simulink model "sf_ttable"  (R2015b)
settings: Solver=ode45  StartTime=0.0  StopTime=10  RelTol=1e-3
settings Model: Creator=amatsumo  LastModifiedBy=amatsumo
settings DataIOCC: SaveFormat=Array  SignalLoggingSaveFormat=ModelDataLogs
settings OptimizationCC: BlockReduction=off  ConditionallyExecuteInputs=off  ExpressionDepthLimit=2147483647
settings DebuggingCC: UnderspecifiedInitializationDetection=Classic  MergeDetectMultiDrivingBlocksExec=none  SolverPrmCheckMsg=warning  FcnCallInpInsideContextMsg=UseLocalSettings  StateNameClashWarn=warning
settings HardwareCC: ProdBitPerPointer=32  ProdLargestAtomicFloat=None  ProdIntDivRoundTo=Undefined  ProdEndianess=Unspecified  ProdWordSize=32  ProdHWDeviceType=32-bit Generic
settings GRTTargetCC: GeneratePreprocessorConditionals=Disable all  CombineOutputUpdateFcns=off  GRTInterface=on
settings ConfigComp: CovMetricSettings=dcw  CovHTMLOptions=-aTS=1 -bRG=1 -bTC=1 -hTR=0 -nFC=0 -scm=1 -bcm=1 -xEv=0  CovNameIncrementing=on  CovSFcnEnable=off

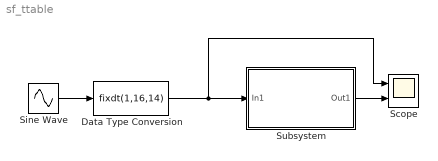
== system sf_ttable ==
  Data Type Conversion : DataTypeConversion  OutDataTypeStr=fixdt(1,16,14)
  Scope : Scope  NumInputPorts=2
  Sine Wave : Sin  Bias=-1  SampleTime=1/1000
  Subsystem : Subsystem
  wires:
  Sine Wave/1 -> Data Type Conversion/1
  Subsystem/1(Out1) -> Scope/2
  Data Type Conversion/1 -> Scope/1, Subsystem/1(In1)

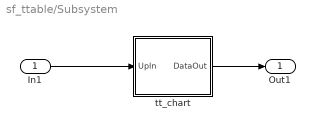
== system sf_ttable/Subsystem ==
  In1 : Inport
  tt_chart : Stateflow chart  TreatAsAtomicUnit=on
  Out1 : Outport
  wires:
  In1/1 -> tt_chart/1(UpIn)
  tt_chart/1(DataOut) -> Out1/1

== stateflow chart sf_ttable/Subsystem/tt_chart ==
  settings: stateMachineType=MEALY_MACHINE  executeAtInitialization=1  initializeOutput=1
  state out = inc_data(in) [function]
    (default) -> (junction 235)
    (junction 235) -> (junction 237) : {
        | /* Positive */
        | aVarTruthTableCondition_1 = (in>1);
        | }
    (junction 237) -> (junction 239) : {
        | /* Negative */
        | aVarTruthTableCondition_2 = ((in>0)&&(in<=1));
        | }
    (junction 239) -> (junction 241) : {
        | /* zero */
        | aVarTruthTableCondition_3 = ((in<=0)&&(in>-1));
        | }
    (junction 241) -> (junction 243) [order 1] : [!aVarTruthTableCondition_1 && !aVarTruthTableCondition_2 && aVarTruthTableCondition_3]
    (junction 243) -> (junction 245) : {
        | /* 'A1':D1 */
        | out = 100
        | }
    (junction 241) -> (junction 247) [order 2]
    (junction 247) -> (junction 249) [order 1] : [!aVarTruthTableCondition_1 && aVarTruthTableCondition_2 && !aVarTruthTableCondition_3]
    (junction 249) -> (junction 251) : {
        | /* 'A2':D2 */
        | out = 10
        | }
    (junction 247) -> (junction 253) [order 2]
    (junction 253) -> (junction 255) [order 1] : [aVarTruthTableCondition_1 && !aVarTruthTableCondition_2 && !aVarTruthTableCondition_3]
    (junction 255) -> (junction 257) : {
        | /* 'A3':D3 */
        | out = 0
        | }
    (junction 253) -> (junction 259) [order 2]
    (junction 259) -> (junction 261) [order 1] : [!aVarTruthTableCondition_1 && !aVarTruthTableCondition_2 && !aVarTruthTableCondition_3]
    (junction 261) -> (junction 263) : {
        | /* 'A4':Else */
        | out = -100
        | }
    (junction 259) -> (junction 265) [order 2]
    (junction 265) -> (junction 267) : /* Default */
    (junction 267) -> (junction 269) : {
        | /* 'A4':Else */
        | out = -100
        | }
  (default) -> (junction 21) : {temp = inc_data(UpIn);
      | DataOut = temp;}
  data: in function_input fixdt(1,16,14); out function_output int16; aVarTruthTableCondition_1 temporary boolean =0; aVarTruthTableCondition_2 temporary boolean =0; aVarTruthTableCondition_3 temporary boolean =0; DataOut output int16; UpIn input fixdt(1,16,14); temp local int16
  data aVarTruthTableCondition_1 settings: description=Positive
  data aVarTruthTableCondition_2 settings: description=Negative
  data aVarTruthTableCondition_3 settings: description=zero
